simulink model "st1"  (R2018b)
settings: Solver=ode45  StartTime=0.0  StopTime=20  RelTol=1e-3
settings Model: Creator=12732  LastModifiedBy=12732
settings DataIOCC: SaveFormat=Array

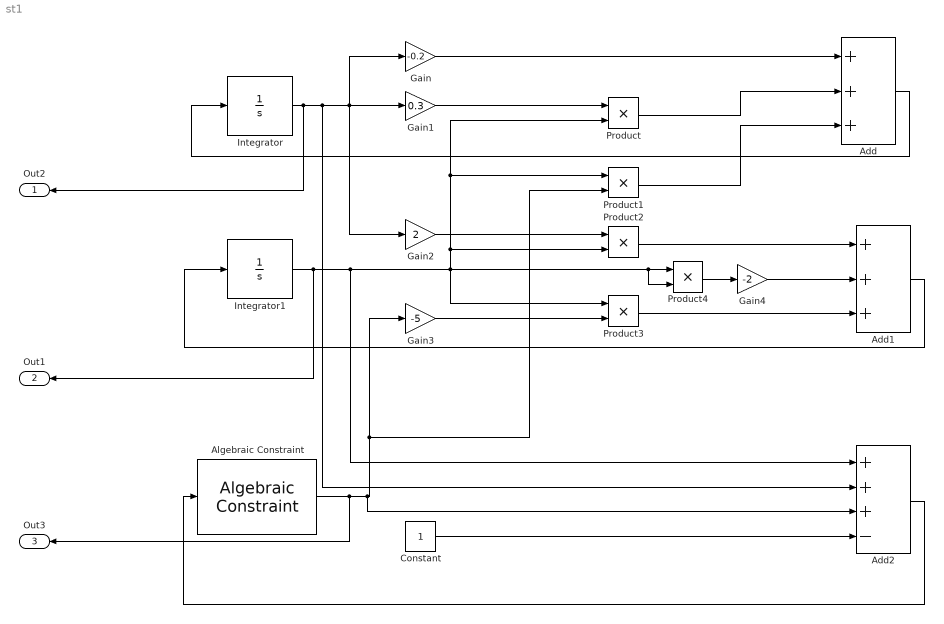
== system st1 ==
  Add : Sum  Inputs=+++
  Add1 : Sum  Inputs=+++
  Add2 : Sum  Inputs=+++-
  Algebraic Constraint : AlgebraicConstraint  InitialGuess=0.1
  Constant : Constant
  Gain : Gain  Gain=-0.2
  Gain1 : Gain  Gain=0.3
  Gain2 : Gain  Gain=2
  Gain3 : Gain  Gain=-5
  Gain4 : Gain  Gain=-2
  Integrator : Integrator  InitialCondition=0.8
  Integrator1 : Integrator  InitialCondition=0.1
  Product{,1..4} (5 alike) : Product
  Out2 : Outport
  Out1 : Outport  Port=2
  Out3 : Outport  Port=3
  wires:
  Integrator/1 -> Out2/1, Add2/2, Gain2/1, Gain/1, Gain1/1
  Gain/1 -> Add/1
  Product/1 -> Add/2
  Product1/1 -> Add/3
  Gain1/1 -> Product/1
  Algebraic Constraint/1 -> Out3/1, Gain3/1, Product1/2, Add2/3
  Gain2/1 -> Product2/1
  Gain3/1 -> Product3/2
  Product2/1 -> Add1/1
  Product3/1 -> Add1/3
  Integrator1/1 -> Out1/1, Add2/1, Product4/2, Product4/1, Product/2, Product1/1, Product2/2, Product3/1
  Product4/1 -> Gain4/1
  Gain4/1 -> Add1/2
  Add1/1 -> Integrator1/1
  Add/1 -> Integrator/1
  Constant/1 -> Add2/4
  Add2/1 -> Algebraic Constraint/1
